simulink model "SimulationANTSMC"  (R2020b)
(part 6 of 18)

                                                                                                                                                                                                                                                                                                                                                                                                                                                                                                                                                                                                                                                                                                                                                                                                                                                                                                                                                                                                                                                                                                                                                                                                                                                                                                                                                                                                                                                                                                                                                                                                                                                                                                                                                                                                                                                                                                                                                                                                                                                                                                                                                                                                                                                                                                                                                                                                                                                                                                                                                                                                                                                                                                                                                                                                                                                                                                                                                                                                                                                                                                                                                                                                                                                                                                                                                                                                                                                                                                                                                                                                                                                                                                                                                                                                                                                                                                                                                                                                                                                                                                                                                                                                                                                                                                                                                                                                                                                                                                                                                                                                                                                                                                                                                                                                                                                                                                                                                                                                                                                                                                                                                                                                                                                                                                                                                                                                                                                                                                                                                                                                                                                                                                                                                                                                                                                                                                                                                                                                                                                                                                                                                                                                                                                                                                                                                                                                                                                                                                                                                                                                                                                                                                                                                                                                                                                                                                                                                                                                                                                                                                                                                                                                                                                                                                                                                                                                                                                                                                                                                                                                                                                                                                                                                                                                                                                                                                                                                                                                                                                                                                                                                                                                                                                                                                                                                                                                                                                                                                                                                                                                                                                                                                                                                                                                                                                                                                                                                                                                                                                                                                                                                                                                                                                                                                                                                                                                                                                                                                                                                                                                                                                                                                                                                                                                                                                                                                                                                                                                                                                                                                                                                                                                                                                                                                                                                                                                                                                                                                                                                                                                                                                                                                                                                                                                                                                                                                                                                                                                                                                                                                                                                                                                                                                                                                                                                                                                                                                                                                                                                                                                                                                                                                                                                                                                                                                                                                                                                                                                                                                                                                                                                                                                                                                                                                                                                                                                                                                                                                                                                                                                                                                                                                                                                                                                                                                                                                                                                                                                                                                                                                                                                                                                                                                                                                                                                                                                                                                                                                                                                                                                                                                                                                                                                                                                                                                                                                                                                                                                                                                                                                                                                                                                                                                                                                                                                                                                                                                                                                                                                                                                                                                                                                                                                                                                                                                                                                                                                                                                                                                                                                                                                                                                                                                                                                                                                                                                                                                                                                                                                                                                                                                                                                                                                                                                                                                                                                                                                                                                                                                                                                                                                                                                                                                                                                                                                                                                                                                                                                                                                                                                                                                                                                                                                                                                                                                                                                                                                                                                                                                                                                                                                                                                                                                                                                                                                                                                                                                                                                                                                                                                                                                                                                                                                                                                                                                                                                                                                                                                                                                                                                                                                                                                                                                                                                                                                                                                                                                                                                                                                                                                                                                                                                                                                                                                                                                                                                                                                                                                                                                                                                                                                                                                                                                                                                                                                                                                                                                                                                                                                                                                                                                                                                                                                                                                                                                                                                                                                                                                                                                                                                                                                                                                                                                                                                                                                                                                                                                                                                                                                                                                                                                                                                                                                                                                                                                                                                                                                                                                                                                                                                                                                                                                                                                                                                                                                                                                                                                                                                                                                                                                                                                                                                                                                                                                                                                                                                                                                                                                                                                                                                                                                                                                                                                                                                                                                                                                                                                                                                                                                                                                                                                                                                                                                                                                                                                                                                                                                                                                                                                                                                                                                                                                                                                                                                                                                                                                                                                                                                                                                                                                                                                                                                                                                                                                                                                                                                                                                                                                                                                                                                                                                                                                                                                                                                                                                                                                                                                                                                                                                                                                                                                                                                                                                                                                                                                                                                                                                                                                                                                                                                                                                                                                                                                                                                                                                                                                                                                                                                                                                                                                                                                                                                                                                                                                                                                                                                                                                                                                                                                                                                                                                                                                                                                                                                                                                                                                                                                                                                                                                                                                                                                                                                                                                                                                                                                                                                                                                                                                                                                                                                                                                                                                                                                                                                                                                                                                                                                                                                                                                                                                                                                                                                                                                                                                                                                                                                                                                                                                                                                                                                                                                                                                                                                                                                                                                                                                                                                                                                                                                                                                                                                                                                                                                                                                                                                                                                                                                                                                                                                                                                                                                                                                                                                                                                                                                                                                                                                                                                                                                                                                                                                                                                                                                                                                                                                                                                                                                                                                                                                                                                                                                                                                                                                                                                                                                                                                                                                                                                                                                                                                                                                                                                                                                                                                                                                                                                                                                                                                                                                                                                                                                                                                                                                                                                                                                                                                                                                                                                                                                                                                                                                                                                                                                                                                                                                                                                                                                                                                                                                                                                                                                                                                                                                                                                                                                                                                                                                                                                                                                                                                                                                                                                                                                                                                                                                                                                                                                                                                                                                                                                                                                                                                                                                                                                                                                                                                                                                                                                                                                                                                                                                                                                                                                                                                                                                                                                                                                                                                                                                                                                                                                                                                                                                                                                                                                                                                                                                                                                                                                                                                                                                                                                                                                                                                                                                                                                                                                                                                                                                                                                                                                                                                                                                                                                                                                                                                                                                                                                                                                                                                                                                                                                                                                                                                                                                                                                                                                                                                                                                                                                                                                                                                                                                                                                                                                                                                                                                                                                                                                                                                                                                                                                                                                                                                                                                                                                                                                                                                                                                                                                                                                                                                                                                                                                                                                                                                                                                                                                                                                                                                                                                                                                                                                                                                                                                                                                                                                                                                                                                                                                                                                                                                                                                                                                                                                                                                                                                                                                                                                                                                                                                                                                                                                                                                                                                                                                                                                                                                                                                                                                                                                                                                                                                                                                                                                                                                                                                                                                                                                                                                                                                                                                                                                                                                                                                                                                                                                                                                                                                                                                                                                                                                                                                                                                                                                                                                                                                                                                                                                                                                                                                                                                                                                                                                                                                                                                                                                                                                                                                                                                                                                                                                                                                                                                                                                                                                                                                                                                                                                                                                                                                                                                                                                                                                                                                                                                                                                                                                                                                                                                                                                                                                                                                                                                                                                                                                                                                                                                                                                                                                                                                                                                                                                                                                                                                                                                                                                                                                                                                                                                                                                                                                                                                                                                                                                                                                                                                                                                                                                                                                                                                                                                                                                                                                                                                                                                                                                                                                                                                                                                                                                                                                                                                                                                                                                                                                                                                                                                                                                                                                                                                                                                                                                                                                                                                                                                                                                                                                                                                                                                                                                                                                                                                                                                                                                                                                                                                                                                                                                                                                                                                                                                                                                                                                                                                                                                                                                                                                                                                                                                                                                                                                                                                                                                                                                                                                                                                                                                                                                                                                                                                                                                                                                                                                                                                                                                                                                                                                                                                                                                                                                                                                                                                                                                                                                                                                                                                                                                                                                                                                                                                                                                                                                                                                                                                                                                                                                                                                                                                                                                                                                                                                                                                                                                                                                                                                                                                                                                                                                                                                                                                                                                                                                                                                                                                                                                                                                                                                                                                                                                                                                                                                                                                                                                                                                                                                                                                                                                                                                                                                                                                                                                                                                                                                                                                                                                                                                                                                                                                                                                                                                                                                                                                                                                                                                                                                                                                                                                                                                                                                                                                                                                                                                                                                                                                                                                                                                                                                                                                                                                                                                                                                                                                                                                                                                                                                                                                                                                                                                                                                                                                                                                                                                                                                                                                                                                                                                                                                                                                                                                                                                                                                                                                                                                                                                                                                                                                                                                                                                                                                                                                                                                                                                                                                                                                                                                                                                                                                                                                                                                                                                                                                                                                                                                                                                                                                                                                                                                                                                                                                                                                                                                                                                                                                                                                                                                                                                                                                                                                                                                                                                                                                                                                                                                                                                                                                                                                                                                                                                                                                                                                                                                                                                                                                                                                                                                                                                                                                                                                                                                                                                                                                                                                                                                                                                                                                                                                                                                                                                                                                                                                                                                                                                                                                                                                                                                                                                                                                                                                                                                                                                                                                                                                                                                                                                                                                                                                                                                                                                                                                                                                                                                                                                                                                                                                                                                                                                                                                                                                                                                                                                                                                                                                                                                                                                                                                                                                                                                                                                                                                                                                                                                                                                                                                                                                                                                                                                                                                                                                                                                                                                                                                                                                                                                                                                                                                                                                                                                                                                                                                                                                                                                                                                                                                                                                                                                                                                                                                                                                                                                                                                                                                                                                                                                                                                                                                                                                                                                                                                                                                                                                                                                                                                                                                                                                                                                                                                                                                                                                                                                                                                                                                                                                                                                                                                                                                                                                                                                                                                                                                                                                                                                                                                                                                                                                                                                                                                                                                                                                                                                                                                                                                                                                                                                                                                                                                                                                                                                                                                                                                                                                                                                                                                                                                                                                                                                                                                                                                                                                                                                                                                                                                                                                                                                                                                                                                                                                                                                                                                                                                                                                                                                                                                                                                                                                                                                                                                                                                                                                                                                                                                                                                                                                                                                                                                                                                                                                                                                                                                                                                                                                                                                                                                                                                                                                                                                                                                                                                                                                                                                                                                                                                                                                                                                                                                                                                                                                                                                                                                                                                                                                                                                                                                                                                                                                                                                                                                                                                                                                                                                                                                                                                                                                                                                                                                                                                                                                                                                                                                                                                                                                                                                                                                                                                                                                                                                                                                                                                                                                                                                                                                                                                                                                                                                                                                                                                                                                                                                                                                                                                                                                                                                                                                                                                                                                                                                                                                                                                                                                                                                                                                                                                                                                                                                                                                                                                                                                                                                                                                                                                                                                                                                                                                                                                                                                                                                                                                                                                                                                                                                                                                                                                                                                                                                                                                                                                                                                                                                                                                                                                                                                                                                                                                                                                               1.96*thetadot2^2*sin(2*theta4) - 1.96*thetadot1^2*sin(2*theta4) - 0.56*thetadot4*thetadot5 + 1.96*thetadot3^2*sin(2*theta4) + 0.12*thetadot2^2*sin(theta3)*sin(theta4) + 0.28*thetadot1^2*sin(theta5)*sin(theta6) - 0.28*thetadot2^2*sin(theta5)*sin(theta6) - 0.28*thetadot3^2*sin(theta5)*sin(theta6) + 0.28*thetadot5^2*sin(theta5)*sin(theta6) - 0.28*thetadot6^2*sin(theta5)*sin(theta6) - 0.56*thetadot4*thetadot5*cos(theta6) + 7.8406*thetadot2*thetadot5*sin(theta4) + 7.8406*thetadot3*thetadot5*sin(theta4) - 0.0801*thetadot5*thetadot6*sin(theta5) + 1.12*thetadot4*thetadot5*cos(theta5)^2 + 3.92*thetadot2*thetadot3*sin(2*theta4) + 3.88*thetadot4*thetadot5*sin(2*theta5) + 0.04*thetadot4*thetadot6*sin(2*theta6) - 0.24*thetadot1*thetadot2*cos(theta4)*sin(theta2) - 0.56*thetadot1*thetadot5*cos(theta2)*sin(theta3) - 0.56*thetadot1*thetadot5*cos(theta3)*sin(theta2) - 0.0801*thetadot2*thetadot6*cos(theta4)*sin(theta5) - 0.0801*thetadot3*thetadot6*cos(theta4)*sin(theta5) - 0.0816*thetadot1*thetadot2*sin(theta2)*sin(theta3) - 0.0816*thetadot1*thetadot3*sin(theta2)*sin(theta3) - 0.56*thetadot2*thetadot3*sin(theta5)*sin(theta6) - 0.56*thetadot2*thetadot6*sin(theta4)*sin(theta6) - 0.56*thetadot3*thetadot6*sin(theta4)*sin(theta6) + 3.92*thetadot1^2*cos(theta2)^2*cos(theta4)*sin(theta4) + 3.92*thetadot1^2*cos(theta3)^2*cos(theta4)*sin(theta4) + 3.88*thetadot1^2*cos(theta4)*cos(theta5)^2*sin(theta4) - 0.04*thetadot1^2*cos(theta4)*cos(theta6)^2*sin(theta4) - 3.88*thetadot2^2*cos(theta4)*cos(theta5)^2*sin(theta4) + 0.04*thetadot2^2*cos(theta4)*cos(theta6)^2*sin(theta4) - 3.88*thetadot3^2*cos(theta4)*cos(theta5)^2*sin(theta4) + 0.04*thetadot3^2*cos(theta4)*cos(theta6)^2*sin(theta4) + 0.12*thetadot1^2*cos(theta2)^2*sin(theta3)*sin(theta4) - 0.28*thetadot1^2*cos(theta2)^2*sin(theta5)*sin(theta6) - 0.28*thetadot1^2*cos(theta3)^2*sin(theta5)*sin(theta6) - 0.56*thetadot1^2*cos(theta4)^2*sin(theta5)*sin(theta6) + 0.56*thetadot2^2*cos(theta4)^2*sin(theta5)*sin(theta6) + 0.56*thetadot3^2*cos(theta4)^2*sin(theta5)*sin(theta6) + 1.12*thetadot4*thetadot5*cos(theta5)^2*cos(theta6) - 7.76*thetadot2*thetadot5*cos(theta5)^2*sin(theta4) - 7.76*thetadot3*thetadot5*cos(theta5)^2*sin(theta4) + 0.08*thetadot5*thetadot6*cos(theta6)^2*sin(theta5) + 0.04*thetadot1^2*cos(theta5)*cos(theta6)*sin(theta6) - 0.04*thetadot2^2*cos(theta5)*cos(theta6)*sin(theta6) - 0.04*thetadot3^2*cos(theta5)*cos(theta6)*sin(theta6) + 0.04*thetadot5^2*cos(theta5)*cos(theta6)*sin(theta6) - 0.26*thetadot1^2*cos(theta2)*sin(theta2)*sin(theta4) - 0.26*thetadot1^2*cos(theta3)*sin(theta3)*sin(theta4) + 0.12*thetadot2^2*cos(theta5)*sin(theta3)*sin(theta4) + 0.12*thetadot2^2*cos(theta4)*sin(theta3)*sin(theta6) + 1.68*thetadot2^2*sin(theta3)*sin(theta4)*sin(theta5) + 0.0816*thetadot1*thetadot2*cos(theta2)*cos(theta3) + 0.0816*thetadot1*thetadot3*cos(theta2)*cos(theta3) - 0.04*thetadot1^2*cos(theta2)^2*cos(theta5)*cos(theta6)*sin(theta6) - 0.04*thetadot1^2*cos(theta3)^2*cos(theta5)*cos(theta6)*sin(theta6) - 0.08*thetadot1^2*cos(theta4)^2*cos(theta5)*cos(theta6)*sin(theta6) + 0.08*thetadot2^2*cos(theta4)^2*cos(theta5)*cos(theta6)*sin(theta6) + 0.08*thetadot3^2*cos(theta4)^2*cos(theta5)*cos(theta6)*sin(theta6) + 0.52*thetadot1^2*cos(theta2)*cos(theta3)^2*sin(theta2)*sin(theta4) + 0.52*thetadot1^2*cos(theta2)^2*cos(theta3)*sin(theta3)*sin(theta4) + 0.56*thetadot1^2*cos(theta2)*cos(theta5)^2*sin(theta2)*sin(theta4) + 0.12*thetadot1^2*cos(theta2)^2*cos(theta5)*sin(theta3)*sin(theta4) + 0.56*thetadot1^2*cos(theta3)*cos(theta5)^2*sin(theta3)*sin(theta4) + 0.12*thetadot1^2*cos(theta2)^2*cos(theta4)*sin(theta3)*sin(theta6) + 1.68*thetadot1^2*cos(theta2)^2*sin(theta3)*sin(theta4)*sin(theta5) + 7.84*thetadot1*thetadot2*cos(theta2)*cos(theta3)*cos(theta4)^2 + 7.84*thetadot1*thetadot3*cos(theta2)*cos(theta3)*cos(theta4)^2 - 0.08*thetadot1*thetadot2*cos(theta2)*cos(theta3)*cos(theta6)^2 - 0.08*thetadot1*thetadot3*cos(theta2)*cos(theta3)*cos(theta6)^2 + 1.12*thetadot1*thetadot5*cos(theta2)*cos(theta5)^2*sin(theta3) + 1.12*thetadot1*thetadot5*cos(theta3)*cos(theta5)^2*sin(theta2) - 7.76*thetadot2*thetadot3*cos(theta4)*cos(theta5)^2*sin(theta4) + 0.08*thetadot2*thetadot3*cos(theta4)*cos(theta6)^2*sin(theta4) + 0.08*thetadot2*thetadot6*cos(theta4)*cos(theta6)^2*sin(theta5) + 0.08*thetadot3*thetadot6*cos(theta4)*cos(theta6)^2*sin(theta5) - 0.08*thetadot4*thetadot5*cos(theta5)*cos(theta6)^2*sin(theta5) - 0.08*thetadot4*thetadot6*cos(theta5)^2*cos(theta6)*sin(theta6) - 7.84*thetadot1*thetadot2*cos(theta4)^2*sin(theta2)*sin(theta3) - 7.84*thetadot1*thetadot3*cos(theta4)^2*sin(theta2)*sin(theta3) + 0.08*thetadot1*thetadot2*cos(theta6)^2*sin(theta2)*sin(theta3) + 0.08*thetadot1*thetadot3*cos(theta6)^2*sin(theta2)*sin(theta3) + 1.12*thetadot2*thetadot3*cos(theta4)^2*sin(theta5)*sin(theta6) + 0.56*thetadot2*thetadot6*cos(theta5)^2*sin(theta4)*sin(theta6) + 0.56*thetadot3*thetadot6*cos(theta5)^2*sin(theta4)*sin(theta6) - 7.84*thetadot1^2*cos(theta2)^2*cos(theta3)^2*cos(theta4)*sin(theta4) - 3.88*thetadot1^2*cos(theta2)^2*cos(theta4)*cos(theta5)^2*sin(theta4) + 0.04*thetadot1^2*cos(theta2)^2*cos(theta4)*cos(theta6)^2*sin(theta4) - 3.88*thetadot1^2*cos(theta3)^2*cos(theta4)*cos(theta5)^2*sin(theta4) + 0.04*thetadot1^2*cos(theta3)^2*cos(theta4)*cos(theta6)^2*sin(theta4) - 0.04*thetadot1^2*cos(theta4)*cos(theta5)^2*cos(theta6)^2*sin(theta4) + 0.04*thetadot2^2*cos(theta4)*cos(theta5)^2*cos(theta6)^2*sin(theta4) + 0.04*thetadot3^2*cos(theta4)*cos(theta5)^2*cos(theta6)^2*sin(theta4) + 0.56*thetadot1^2*cos(theta2)^2*cos(theta3)^2*sin(theta5)*sin(theta6) + 0.56*thetadot1^2*cos(theta2)^2*cos(theta4)^2*sin(theta5)*sin(theta6) + 0.56*thetadot1^2*cos(theta3)^2*cos(theta4)^2*sin(theta5)*sin(theta6) + 0.08*thetadot2*thetadot5*cos(theta5)^2*cos(theta6)^2*sin(theta4) + 0.08*thetadot3*thetadot5*cos(theta5)^2*cos(theta6)^2*sin(theta4) + 0.12*thetadot1^2*cos(theta2)*cos(theta3)*sin(theta2)*sin(theta4) - 0.3*thetadot1^2*cos(theta2)*cos(theta5)*sin(theta2)*sin(theta4) - 0.3*thetadot1^2*cos(theta2)*cos(theta4)*sin(theta2)*sin(theta6) - 0.28*thetadot1^2*cos(theta2)*cos(theta6)*sin(theta2)*sin(theta4) - 0.3*thetadot1^2*cos(theta3)*cos(theta5)*sin(theta3)*sin(theta4) - 0.3*thetadot1^2*cos(theta3)*cos(theta4)*sin(theta3)*sin(theta6) - 0.28*thetadot1^2*cos(theta3)*cos(theta6)*sin(theta3)*sin(theta4) - 0.56*thetadot1^2*cos(theta4)*cos(theta5)*sin(theta4)*sin(theta5) + 0.56*thetadot2^2*cos(theta4)*cos(theta5)*sin(theta4)*sin(theta5) + 0.12*thetadot2^2*cos(theta5)*cos(theta6)*sin(theta3)*sin(theta4) + 0.56*thetadot3^2*cos(theta4)*cos(theta5)*sin(theta4)*sin(theta5) - 4.2*thetadot1^2*cos(theta2)*sin(theta2)*sin(theta4)*sin(theta5) - 4.2*thetadot1^2*cos(theta3)*sin(theta3)*sin(theta4)*sin(theta5) + 7.8406*thetadot1*thetadot5*cos(theta2)*cos(theta3)*cos(theta4) - 0.52*thetadot1*thetadot2*cos(theta2)*cos(theta4)*sin(theta3) - 0.52*thetadot1*thetadot2*cos(theta3)*cos(theta4)*sin(theta2) - 0.52*thetadot1*thetadot3*cos(theta2)*cos(theta4)*sin(theta3) - 0.52*thetadot1*thetadot3*cos(theta3)*cos(theta4)*sin(theta2) - 0.24*thetadot1*thetadot2*cos(theta4)*cos(theta5)*sin(theta2) + 1.041784545864672835129637359261e-36*thetadot1*thetadot4*cos(theta2)*cos(theta3)*sin(theta4) - 0.56*thetadot1*thetadot5*cos(theta2)*cos(theta6)*sin(theta3) - 0.56*thetadot1*thetadot5*cos(theta3)*cos(theta6)*sin(theta2) - 0.08*thetadot2*thetadot3*cos(theta5)*cos(theta6)*sin(theta6) - 3.36*thetadot1*thetadot2*cos(theta4)*sin(theta2)*sin(theta5) + 4.4200467277063457510618654694995e-35*thetadot1*thetadot4*cos(theta2)*sin(theta3)*sin(theta4) + 4.4200467277063457510618654694995e-35*thetadot1*thetadot4*cos(theta3)*sin(theta2)*sin(theta4) - 7.8406*thetadot1*thetadot5*cos(theta4)*sin(theta2)*sin(theta3) + 1.12*thetadot2*thetadot5*cos(theta5)*sin(theta4)*sin(theta5) + 0.56*thetadot2*thetadot5*cos(theta4)*sin(theta5)*sin(theta6) + 1.12*thetadot3*thetadot5*cos(theta5)*sin(theta4)*sin(theta5) + 0.56*thetadot3*thetadot5*cos(theta4)*sin(theta5)*sin(theta6) - 0.56*thetadot4*thetadot6*cos(theta5)*sin(theta5)*sin(theta6) - 1.041784545864672835129637359261e-36*thetadot1*thetadot4*sin(theta2)*sin(theta3)*sin(theta4) + 0.24*thetadot1*thetadot2*sin(theta2)*sin(theta4)*sin(theta6) - 7.76*thetadot1*thetadot5*cos(theta2)*cos(theta3)*cos(theta4)*cos(theta5)^2 + 1.12*thetadot1*thetadot2*cos(theta2)*cos(theta4)*cos(theta5)^2*sin(theta3) + 1.12*thetadot1*thetadot2*cos(theta3)*cos(theta4)*cos(theta5)^2*sin(theta2) + 1.12*thetadot1*thetadot3*cos(theta2)*cos(theta4)*cos(theta5)^2*sin(theta3) + 1.12*thetadot1*thetadot3*cos(theta3)*cos(theta4)*cos(theta5)^2*sin(theta2) + 1.12*thetadot1*thetadot5*cos(theta2)*cos(theta5)^2*cos(theta6)*sin(theta3) + 1.12*thetadot1*thetadot5*cos(theta3)*cos(theta5)^2*cos(theta6)*sin(theta2) + 0.16*thetadot2*thetadot3*cos(theta4)^2*cos(theta5)*cos(theta6)*sin(theta6) + 7.76*thetadot1*thetadot5*cos(theta4)*cos(theta5)^2*sin(theta2)*sin(theta3) + 0.08*thetadot1^2*cos(theta2)^2*cos(theta3)^2*cos(theta5)*cos(theta6)*sin(theta6) + 0.08*thetadot1^2*cos(theta2)^2*cos(theta4)^2*cos(theta5)*cos(theta6)*sin(theta6) + 0.08*thetadot1^2*cos(theta3)^2*cos(theta4)^2*cos(theta5)*cos(theta6)*sin(theta6) - 1.12*thetadot1^2*cos(theta2)*cos(theta3)^2*cos(theta5)^2*sin(theta2)*sin(theta4) - 1.12*thetadot1^2*cos(theta2)^2*cos(theta3)*cos(theta5)^2*sin(theta3)*sin(theta4) - 7.76*thetadot1*thetadot2*cos(theta2)*cos(theta3)*cos(theta4)^2*cos(theta5)^2 + 0.08*thetadot1*thetadot2*cos(theta2)*cos(theta3)*cos(theta4)^2*cos(theta6)^2 - 7.76*thetadot1*thetadot3*cos(theta2)*cos(theta3)*cos(theta4)^2*cos(theta5)^2 + 0.08*thetadot1*thetadot3*cos(theta2)*cos(theta3)*cos(theta4)^2*cos(theta6)^2 + 0.08*thetadot2*thetadot3*cos(theta4)*cos(theta5)^2*cos(theta6)^2*sin(theta4) + 7.76*thetadot1*thetadot2*cos(theta4)^2*cos(theta5)^2*sin(theta2)*sin(theta3) - 0.08*thetadot1*thetadot2*cos(theta4)^2*cos(theta6)^2*sin(theta2)*sin(theta3) + 7.76*thetadot1*thetadot3*cos(theta4)^2*cos(theta5)^2*sin(theta2)*sin(theta3) - 0.08*thetadot1*thetadot3*cos(theta4)^2*cos(theta6)^2*sin(theta2)*sin(theta3) + 0.12*thetadot1^2*cos(theta2)*cos(theta3)*cos(theta5)*sin(theta2)*sin(theta4) + 0.12*thetadot1^2*cos(theta2)*cos(theta3)*cos(theta4)*sin(theta2)*sin(theta6) + 0.28*thetadot1^2*cos(theta2)*cos(theta4)*cos(theta5)*sin(theta2)*sin(theta6) - 0.3*thetadot1^2*cos(theta2)*cos(theta5)*cos(theta6)*sin(theta2)*sin(theta4) + 0.28*thetadot1^2*cos(theta3)*cos(theta4)*cos(theta5)*sin(theta3)*sin(theta6) - 0.3*thetadot1^2*cos(theta3)*cos(theta5)*cos(theta6)*sin(theta3)*sin(theta4) - 0.56*thetadot1^2*cos(theta4)*cos(theta5)*cos(theta6)*sin(theta4)*sin(theta5) + 0.56*thetadot2^2*cos(theta4)*cos(theta5)*cos(theta6)*sin(theta4)*sin(theta5) + 0.56*thetadot3^2*cos(theta4)*cos(theta5)*cos(theta6)*sin(theta4)*sin(theta5) + 7.76*thetadot1^2*cos(theta2)^2*cos(theta3)^2*cos(theta4)*cos(theta5)^2*sin(theta4) - 0.08*thetadot1^2*cos(theta2)^2*cos(theta3)^2*cos(theta4)*cos(theta6)^2*sin(theta4) + 0.04*thetadot1^2*cos(theta2)^2*cos(theta4)*cos(theta5)^2*cos(theta6)^2*sin(theta4) + 0.04*thetadot1^2*cos(theta3)^2*cos(theta4)*cos(theta5)^2*cos(theta6)^2*sin(theta4) + 1.68*thetadot1^2*cos(theta2)*cos(theta3)*sin(theta2)*sin(theta4)*sin(theta5) + 3.88*thetadot1^2*cos(theta2)*cos(theta5)*sin(theta2)*sin(theta4)*sin(theta5) + 3.88*thetadot1^2*cos(theta3)*cos(theta5)*sin(theta3)*sin(theta4)*sin(theta5) - 1.12*thetadot1^2*cos(theta2)^2*cos(theta3)^2*cos(theta4)^2*sin(theta5)*sin(theta6) - 0.6*thetadot1*thetadot2*cos(theta2)*cos(theta4)*cos(theta5)*sin(theta3) - 0.6*thetadot1*thetadot2*cos(theta3)*cos(theta4)*cos(theta5)*sin(theta2) - 0.56*thetadot1*thetadot2*cos(theta2)*cos(theta4)*cos(theta6)*sin(theta3) - 0.56*thetadot1*thetadot2*cos(theta3)*cos(theta4)*cos(theta6)*sin(theta2) - 0.6*thetadot1*thetadot3*cos(theta2)*cos(theta4)*cos(theta5)*sin(theta3) - 0.6*thetadot1*thetadot3*cos(theta3)*cos(theta4)*cos(theta5)*sin(theta2) - 0.56*thetadot1*thetadot3*cos(theta2)*cos(theta4)*cos(theta6)*sin(theta3) - 0.56*thetadot1*thetadot3*cos(theta3)*cos(theta4)*cos(theta6)*sin(theta2) - 0.24*thetadot1*thetadot2*cos(theta4)*cos(theta5)*cos(theta6)*sin(theta2) - 0.56*thetadot1*thetadot6*cos(theta2)*cos(theta3)*cos(theta4)*sin(theta6) + 0.08*thetadot2*thetadot5*cos(theta4)*cos(theta5)*cos(theta6)*sin(theta6) + 0.08*thetadot3*thetadot5*cos(theta4)*cos(theta5)*cos(theta6)*sin(theta6) - 8.4*thetadot1*thetadot2*cos(theta2)*cos(theta4)*sin(theta3)*sin(theta5) - 8.4*thetadot1*thetadot2*cos(theta3)*cos(theta4)*sin(theta2)*sin(theta5) - 8.4*thetadot1*thetadot3*cos(theta2)*cos(theta4)*sin(theta3)*sin(theta5) - 8.4*thetadot1*thetadot3*cos(theta3)*cos(theta4)*sin(theta2)*sin(theta5) + 4.4200467277063457510618654694995e-35*thetadot1*thetadot4*cos(theta2)*cos(theta5)*sin(theta3)*sin(theta4) + 4.4200467277063457510618654694995e-35*thetadot1*thetadot4*cos(theta3)*cos(theta5)*sin(theta2)*sin(theta4) + 4.4200467277063457510618654694995e-35*thetadot1*thetadot4*cos(theta2)*cos(theta4)*sin(theta3)*sin(theta6) + 4.4200467277063457510618654694995e-35*thetadot1*thetadot4*cos(theta3)*cos(theta4)*sin(theta2)*sin(theta6) + 7.76*thetadot1*thetadot5*cos(theta2)*cos(theta5)*sin(theta3)*sin(theta5) + 7.76*thetadot1*thetadot5*cos(theta3)*cos(theta5)*sin(theta2)*sin(theta5) + 0.0801*thetadot1*thetadot6*cos(theta2)*cos(theta3)*sin(theta4)*sin(theta5) + 1.12*thetadot2*thetadot3*cos(theta4)*cos(theta5)*sin(theta4)*sin(theta5) + 0.08*thetadot1*thetadot6*cos(theta2)*cos(theta6)*sin(theta3)*sin(theta6) + 0.08*thetadot1*thetadot6*cos(theta3)*cos(theta6)*sin(theta2)*sin(theta6) + 1.12*thetadot2*thetadot5*cos(theta5)*cos(theta6)*sin(theta4)*sin(theta5) + 1.12*thetadot3*thetadot5*cos(theta5)*cos(theta6)*sin(theta4)*sin(theta5) + 0.6*thetadot1*thetadot2*cos(theta2)*sin(theta3)*sin(theta4)*sin(theta6) + 0.6*thetadot1*thetadot2*cos(theta3)*sin(theta2)*sin(theta4)*sin(theta6) + 0.6*thetadot1*thetadot3*cos(theta2)*sin(theta3)*sin(theta4)*sin(theta6) + 0.6*thetadot1*thetadot3*cos(theta3)*sin(theta2)*sin(theta4)*sin(theta6) + 6.1880654187888840514866116572993e-34*thetadot1*thetadot4*cos(theta2)*sin(theta3)*sin(theta4)*sin(theta5) + 6.1880654187888840514866116572993e-34*thetadot1*thetadot4*cos(theta3)*sin(theta2)*sin(theta4)*sin(theta5) + 0.56*thetadot1*thetadot6*cos(theta4)*sin(theta2)*sin(theta3)*sin(theta6) - 0.0801*thetadot1*thetadot6*sin(theta2)*sin(theta3)*sin(theta4)*sin(theta5) + 0.6*thetadot1^2*cos(theta2)*cos(theta3)^2*cos(theta5)*sin(theta2)*sin(theta4) + 0.6*thetadot1^2*cos(theta2)*cos(theta3)^2*cos(theta4)*sin(theta2)*sin(theta6) + 0.56*thetadot1^2*cos(theta2)*cos(theta3)^2*cos(theta6)*sin(theta2)*sin(theta4) + 0.6*thetadot1^2*cos(theta2)^2*cos(theta3)*cos(theta5)*sin(theta3)*sin(theta4) + 0.6*thetadot1^2*cos(theta2)^2*cos(theta3)*cos(theta4)*sin(theta3)*sin(theta6) + 0.56*thetadot1^2*cos(theta2)^2*cos(theta3)*cos(theta6)*sin(theta3)*sin(theta4) + 0.56*thetadot1^2*cos(theta2)*cos(theta5)^2*cos(theta6)*sin(theta2)*sin(theta4) + 0.56*thetadot1^2*cos(theta2)^2*cos(theta4)*cos(theta5)*sin(theta4)*sin(theta5) + 0.12*thetadot1^2*cos(theta2)^2*cos(theta5)*cos(theta6)*sin(theta3)*sin(theta4) + 0.56*thetadot1^2*cos(theta3)*cos(theta5)^2*cos(theta6)*sin(theta3)*sin(theta4) + 0.56*thetadot1^2*cos(theta3)^2*cos(theta4)*cos(theta5)*sin(theta4)*sin(theta5) + 8.4*thetadot1^2*cos(theta2)*cos(theta3)^2*sin(theta2)*sin(theta4)*sin(theta5) + 8.4*thetadot1^2*cos(theta2)^2*cos(theta3)*sin(theta3)*sin(theta4)*sin(theta5) - 1.12*thetadot1*thetadot2*cos(theta4)^2*cos(theta5)*sin(theta2)*sin(theta3)*sin(theta5) - 1.12*thetadot1*thetadot3*cos(theta4)^2*cos(theta5)*sin(theta2)*sin(theta3)*sin(theta5) - 1.041784545864672835129637359261e-36*thetadot1*thetadot4*cos(theta4)*cos(theta5)^2*sin(theta2)*sin(theta3)*sin(theta6) - 0.56*thetadot1*thetadot6*cos(theta4)*cos(theta5)^2*sin(theta2)*sin(theta3)*sin(theta6) + 0.08*thetadot1*thetadot6*cos(theta6)^2*sin(theta2)*sin(theta3)*sin(theta4)*sin(theta5) - 1.12*thetadot1^2*cos(theta2)*cos(theta3)^2*cos(theta5)^2*cos(theta6)*sin(theta2)*sin(theta4) - 1.12*thetadot1^2*cos(theta2)^2*cos(theta3)*cos(theta5)^2*cos(theta6)*sin(theta3)*sin(theta4) - 1.12*thetadot1^2*cos(theta2)^2*cos(theta3)^2*cos(theta4)*cos(theta5)*sin(theta4)*sin(theta5) + 0.08*thetadot1*thetadot5*cos(theta2)*cos(theta3)*cos(theta4)*cos(theta5)^2*cos(theta6)^2 - 0.08*thetadot1*thetadot5*cos(theta4)*cos(theta5)^2*cos(theta6)^2*sin(theta2)*sin(theta3) + 0.12*thetadot1^2*cos(theta2)*cos(theta3)*cos(theta5)*cos(theta6)*sin(theta2)*sin(theta4) - 0.16*thetadot1^2*cos(theta2)^2*cos(theta3)^2*cos(theta4)^2*cos(theta5)*cos(theta6)*sin(theta6) + 7.84*thetadot1^2*cos(theta2)*cos(theta3)*cos(theta4)*sin(theta2)*sin(theta3)*sin(theta4) - 0.04*thetadot1^2*cos(theta2)*cos(theta4)*cos(theta6)*sin(theta2)*sin(theta5)*sin(theta6) - 0.04*thetadot1^2*cos(theta3)*cos(theta4)*cos(theta6)*sin(theta3)*sin(theta5)*sin(theta6) - 0.56*thetadot1^2*cos(theta2)*cos(theta3)*sin(theta2)*sin(theta3)*sin(theta5)*sin(theta6) - 0.6*thetadot1*thetadot2*cos(theta2)*cos(theta4)*cos(theta5)*cos(theta6)*sin(theta3) - 0.6*thetadot1*thetadot2*cos(theta3)*cos(theta4)*cos(theta5)*cos(theta6)*sin(theta2) - 0.6*thetadot1*thetadot3*cos(theta2)*cos(theta4)*cos(theta5)*cos(theta6)*sin(theta3) - 0.6*thetadot1*thetadot3*cos(theta3)*cos(theta4)*cos(theta5)*cos(theta6)*sin(theta2) + 1.12*thetadot1*thetadot5*cos(theta2)*cos(theta3)*cos(theta4)*cos(theta5)*sin(theta5) + 0.08*thetadot1*thetadot2*cos(theta2)*cos(theta3)*cos(theta4)^2*cos(theta5)^2*cos(theta6)^2 + 0.08*thetadot1*thetadot3*cos(theta2)*cos(theta3)*cos(theta4)^2*cos(theta5)^2*cos(theta6)^2 + 7.76*thetadot1*thetadot2*cos(theta2)*cos(theta4)*cos(theta5)*sin(theta3)*sin(theta5) + 7.76*thetadot1*thetadot2*cos(theta3)*cos(theta4)*cos(theta5)*sin(theta2)*sin(theta5) + 7.76*thetadot1*thetadot3*cos(theta2)*cos(theta4)*cos(theta5)*sin(theta3)*sin(theta5) + 7.76*thetadot1*thetadot3*cos(theta3)*cos(theta4)*cos(theta5)*sin(theta2)*sin(theta5) + 4.4200467277063457510618654694995e-35*thetadot1*thetadot4*cos(theta2)*cos(theta5)*cos(theta6)*sin(theta3)*sin(theta4) + 4.4200467277063457510618654694995e-35*thetadot1*thetadot4*cos(theta3)*cos(theta5)*cos(theta6)*sin(theta2)*sin(theta4) + 1.12*thetadot2*thetadot3*cos(theta4)*cos(theta5)*cos(theta6)*sin(theta4)*sin(theta5) - 0.56*thetadot1*thetadot2*cos(theta2)*cos(theta5)*sin(theta3)*sin(theta4)*sin(theta6) - 0.56*thetadot1*thetadot2*cos(theta3)*cos(theta5)*sin(theta2)*sin(theta4)*sin(theta6) - 0.56*thetadot1*thetadot3*cos(theta2)*cos(theta5)*sin(theta3)*sin(theta4)*sin(theta6) - 0.56*thetadot1*thetadot3*cos(theta3)*cos(theta5)*sin(theta2)*sin(theta4)*sin(theta6) - 1.12*thetadot1*thetadot5*cos(theta4)*cos(theta5)*sin(theta2)*sin(theta3)*sin(theta5) - 0.56*thetadot1*thetadot5*cos(theta2)*cos(theta3)*sin(theta4)*sin(theta5)*sin(theta6) - 0.56*thetadot1*thetadot6*cos(theta2)*cos(theta5)*sin(theta3)*sin(theta5)*sin(theta6) - 0.56*thetadot1*thetadot6*cos(theta3)*cos(theta5)*sin(theta2)*sin(theta5)*sin(theta6) - 0.08*thetadot2*thetadot6*cos(theta5)*cos(theta6)*sin(theta4)*sin(theta5)*sin(theta6) - 0.08*thetadot3*thetadot6*cos(theta5)*cos(theta6)*sin(theta4)*sin(theta5)*sin(theta6) - 0.08*thetadot1*thetadot2*cos(theta4)^2*cos(theta5)^2*cos(theta6)^2*sin(theta2)*sin(theta3) - 0.08*thetadot1*thetadot3*cos(theta4)^2*cos(theta5)^2*cos(theta6)^2*sin(theta2)*sin(theta3) - 0.56*thetadot1^2*cos(theta2)*cos(theta3)^2*cos(theta4)*cos(theta5)*sin(theta2)*sin(theta6) + 0.6*thetadot1^2*cos(theta2)*cos(theta3)^2*cos(theta5)*cos(theta6)*sin(theta2)*sin(theta4) - 0.56*thetadot1^2*cos(theta2)^2*cos(theta3)*cos(theta4)*cos(theta5)*sin(theta3)*sin(theta6) + 0.6*thetadot1^2*cos(theta2)^2*cos(theta3)*cos(theta5)*cos(theta6)*sin(theta3)*sin(theta4) + 0.56*thetadot1^2*cos(theta2)^2*cos(theta4)*cos(theta5)*cos(theta6)*sin(theta4)*sin(theta5) + 0.56*thetadot1^2*cos(theta3)^2*cos(theta4)*cos(theta5)*cos(theta6)*sin(theta4)*sin(theta5) + 0.56*thetadot1*thetadot5*sin(theta2)*sin(theta3)*sin(theta4)*sin(theta5)*sin(theta6) - 0.08*thetadot1^2*cos(theta2)^2*cos(theta3)^2*cos(theta4)*cos(theta5)^2*cos(theta6)^2*sin(theta4) - 7.76*thetadot1^2*cos(theta2)*cos(theta3)^2*cos(theta5)*sin(theta2)*sin(theta4)*sin(theta5) - 7.76*thetadot1^2*cos(theta2)^2*cos(theta3)*cos(theta5)*sin(theta3)*sin(theta4)*sin(theta5) - 0.04*thetadot1^2*cos(theta2)*cos(theta5)*cos(theta6)^2*sin(theta2)*sin(theta4)*sin(theta5) - 0.04*thetadot1^2*cos(theta3)*cos(theta5)*cos(theta6)^2*sin(theta3)*sin(theta4)*sin(theta5) + 1.12*thetadot1*thetadot2*cos(theta2)*cos(theta3)*cos(theta4)^2*cos(theta5)*sin(theta5) + 1.12*thetadot1*thetadot2*cos(theta2)*cos(theta4)*cos(theta5)^2*cos(theta6)*sin(theta3) + 1.12*thetadot1*thetadot2*cos(theta3)*cos(theta4)*cos(theta5)^2*cos(theta6)*sin(theta2) + 1.12*thetadot1*thetadot3*cos(theta2)*cos(theta3)*cos(theta4)^2*cos(theta5)*sin(theta5) + 1.12*thetadot1*thetadot3*cos(theta2)*cos(theta4)*cos(theta5)^2*cos(theta6)*sin(theta3) + 1.12*thetadot1*thetadot3*cos(theta3)*cos(theta4)*cos(theta5)^2*cos(theta6)*sin(theta2) + 1.041784545864672835129637359261e-36*thetadot1*thetadot4*cos(theta2)*cos(theta3)*cos(theta4)*cos(theta5)^2*sin(theta6) + 0.56*thetadot1*thetadot6*cos(theta2)*cos(theta3)*cos(theta4)*cos(theta5)^2*sin(theta6) - 0.08*thetadot1*thetadot5*cos(theta2)*cos(theta5)*cos(theta6)^2*sin(theta3)*sin(theta5) - 0.08*thetadot1*thetadot5*cos(theta3)*cos(theta5)*cos(theta6)^2*sin(theta2)*sin(theta5) - 0.08*thetadot1*thetadot6*cos(theta2)*cos(theta3)*cos(theta6)^2*sin(theta4)*sin(theta5) - 0.08*thetadot1*thetadot6*cos(theta2)*cos(theta5)^2*cos(theta6)*sin(theta3)*sin(theta6) - 0.08*thetadot1*thetadot6*cos(theta3)*cos(theta5)^2*cos(theta6)*sin(theta2)*sin(theta6) + 0.08*thetadot1^2*cos(theta2)*cos(theta3)^2*cos(theta5)*cos(theta6)^2*sin(theta2)*sin(theta4)*sin(theta5) + 0.08*thetadot1^2*cos(theta2)^2*cos(theta3)*cos(theta5)*cos(theta6)^2*sin(theta3)*sin(theta4)*sin(theta5) - 0.08*thetadot1^2*cos(theta2)*cos(theta3)*cos(theta5)*cos(theta6)*sin(theta2)*sin(theta3)*sin(theta6) + 1.12*thetadot1*thetadot5*cos(theta2)*cos(theta3)*cos(theta4)*cos(theta5)*cos(theta6)*sin(theta5) - 0.08*thetadot1*thetadot5*cos(theta2)*cos(theta3)*cos(theta5)*cos(theta6)*sin(theta4)*sin(theta6) - 1.12*thetadot1*thetadot2*cos(theta2)*cos(theta3)*cos(theta4)*sin(theta4)*sin(theta5)*sin(theta6) - 1.12*thetadot1*thetadot3*cos(theta2)*cos(theta3)*cos(theta4)*sin(theta4)*sin(theta5)*sin(theta6) - 1.12*thetadot1*thetadot5*cos(theta4)*cos(theta5)*cos(theta6)*sin(theta2)*sin(theta3)*sin(theta5) + 0.08*thetadot1*thetadot2*cos(theta2)*cos(theta6)*sin(theta3)*sin(theta4)*sin(theta5)*sin(theta6) + 0.08*thetadot1*thetadot2*cos(theta3)*cos(theta6)*sin(theta2)*sin(theta4)*sin(theta5)*sin(theta6) + 0.08*thetadot1*thetadot3*cos(theta2)*cos(theta6)*sin(theta3)*sin(theta4)*sin(theta5)*sin(theta6) + 0.08*thetadot1*thetadot3*cos(theta3)*cos(theta6)*sin(theta2)*sin(theta4)*sin(theta5)*sin(theta6) + 0.08*thetadot1*thetadot5*cos(theta5)*cos(theta6)*sin(theta2)*sin(theta3)*sin(theta4)*sin(theta6) + 1.12*thetadot1*thetadot2*cos(theta4)*sin(theta2)*sin(theta3)*sin(theta4)*sin(theta5)*sin(theta6) + 1.12*thetadot1*thetadot3*cos(theta4)*sin(theta2)*sin(theta3)*sin(theta4)*sin(theta5)*sin(theta6) - 7.76*thetadot1^2*cos(theta2)*cos(theta3)*cos(theta4)*cos(theta5)^2*sin(theta2)*sin(theta3)*sin(theta4) + 0.08*thetadot1^2*cos(theta2)*cos(theta3)*cos(theta4)*cos(theta6)^2*sin(theta2)*sin(theta3)*sin(theta4) + 0.08*thetadot1^2*cos(theta2)*cos(theta3)^2*cos(theta4)*cos(theta6)*sin(theta2)*sin(theta5)*sin(theta6) + 0.08*thetadot1^2*cos(theta2)^2*cos(theta3)*cos(theta4)*cos(theta6)*sin(theta3)*sin(theta5)*sin(theta6) + 1.12*thetadot1^2*cos(theta2)*cos(theta3)*cos(theta4)^2*sin(theta2)*sin(theta3)*sin(theta5)*sin(theta6) + 1.12*thetadot1*thetadot2*cos(theta2)*cos(theta3)*cos(theta4)^2*cos(theta5)*cos(theta6)*sin(theta5) + 1.12*thetadot1*thetadot3*cos(theta2)*cos(theta3)*cos(theta4)^2*cos(theta5)*cos(theta6)*sin(theta5) - 0.08*thetadot1*thetadot2*cos(theta2)*cos(theta4)*cos(theta5)*cos(theta6)^2*sin(theta3)*sin(theta5) - 0.08*thetadot1*thetadot2*cos(theta3)*cos(theta4)*cos(theta5)*cos(theta6)^2*sin(theta2)*sin(theta5) - 0.08*thetadot1*thetadot3*cos(theta2)*cos(theta4)*cos(theta5)*cos(theta6)^2*sin(theta3)*sin(theta5) - 0.08*thetadot1*thetadot3*cos(theta3)*cos(theta4)*cos(theta5)*cos(theta6)^2*sin(theta2)*sin(theta5) - 1.12*thetadot1*thetadot2*cos(theta4)^2*cos(theta5)*cos(theta6)*sin(theta2)*sin(theta3)*sin(theta5) - 1.12*thetadot1*thetadot3*cos(theta4)^2*cos(theta5)*cos(theta6)*sin(theta2)*sin(theta3)*sin(theta5) - 1.12*thetadot1^2*cos(theta2)^2*cos(theta3)^2*cos(theta4)*cos(theta5)*cos(theta6)*sin(theta4)*sin(theta5) + 1.12*thetadot1^2*cos(theta2)*cos(theta3)*cos(theta4)*cos(theta5)*sin(theta2)*sin(theta3)*sin(theta4)*sin(theta5) - 0.16*thetadot1*thetadot2*cos(theta2)*cos(theta3)*cos(theta4)*cos(theta5)*cos(theta6)*sin(theta4)*sin(theta6) - 0.16*thetadot1*thetadot3*cos(theta2)*cos(theta3)*cos(theta4)*cos(theta5)*cos(theta6)*sin(theta4)*sin(theta6) - 0.08*thetadot1*thetadot6*cos(theta2)*cos(theta3)*cos(theta4)*cos(theta5)*cos(theta6)*sin(theta5)*sin(theta6) + 0.16*thetadot1*thetadot2*cos(theta4)*cos(theta5)*cos(theta6)*sin(theta2)*sin(theta3)*sin(theta4)*sin(theta6) + 0.16*thetadot1*thetadot3*cos(theta4)*cos(theta5)*cos(theta6)*sin(theta2)*sin(theta3)*sin(theta4)*sin(theta6) + 0.08*thetadot1*thetadot6*cos(theta4)*cos(theta5)*cos(theta6)*sin(theta2)*sin(theta3)*sin(theta5)*sin(theta6) + 0.16*thetadot1^2*cos(theta2)*cos(theta3)*cos(theta4)^2*cos(theta5)*cos(theta6)*sin(theta2)*sin(theta3)*sin(theta6) + 0.08*thetadot1^2*cos(theta2)*cos(theta3)*cos(theta4)*cos(theta5)^2*cos(theta6)^2*sin(theta2)*sin(theta3)*sin(theta4) + 1.12*thetadot1^2*cos(theta2)*cos(theta3)*cos(theta4)*cos(theta5)*cos(theta6)*sin(theta2)*sin(theta3)*sin(theta4)*sin(theta5);
